simulink model "controller_dev_py"  (R2018b)
settings: Solver=ode2  StartTime=0.0  StopTime=inf  FixedStep=tS  RelTol=1e-3  EnableMultiTasking=on
model workspace (MAT data in the model file):
  m = 1000
settings Model: DataDictionary=controller_dev_py.sldd  PauseTimes=6.42  Creator=wischnewski  LastModifiedBy=ge34qer
settings DataIOCC: SaveOutput=off  SignalLogging=off  DSMLogging=off  SaveTime=off
settings OptimizationCC: StrengthReduction=on  PassReuseOutputArgsAs=Individual arguments  OptimizeBlockOrder=speed  OptimizationPriority=Speed  OptimizationCustomize=off
settings DebuggingCC: UnderspecifiedInitializationDetection=Classic  MergeDetectMultiDrivingBlocksExec=none  ParameterTunabilityLossMsg=error
settings ModelReferenceCC: PropagateSignalLabelsOutOfModel=off
settings SFSimCC: MATLABDynamicMemAlloc=off
settings RTWCC: SystemTargetFile=ert.tlc  GenCodeOnly=on  PackageGeneratedCodeAndArtifacts=on  PackageName=controller_dev_py  TemplateMakefile=ert_default_tmf  IncludeHyperlinkInReport=on  TargetLang=C++
settings CodeAppCC: ForceParamTrailComments=on  IgnoreCustomStorageClasses=off  MaxIdLength=64  OperatorAnnotations=on  SimulinkDataObjDesc=on  SFDataObjDesc=on  InsertBlockDesc=on
settings ERTTargetCC: TargetLangStandard=C++03 (ISO)  GenerateSampleERTMain=on  MultiInstanceERTCode=on  CodeInterfacePackaging=Reusable function  SupportContinuousTime=on  SupportVariableSizeSignals=on  GenerateAllocFcn=on  RootIOFormat=Part of model data structure  RTWCAPIParams=on  ERTCustomFileTemplate=example_file_process.tlc

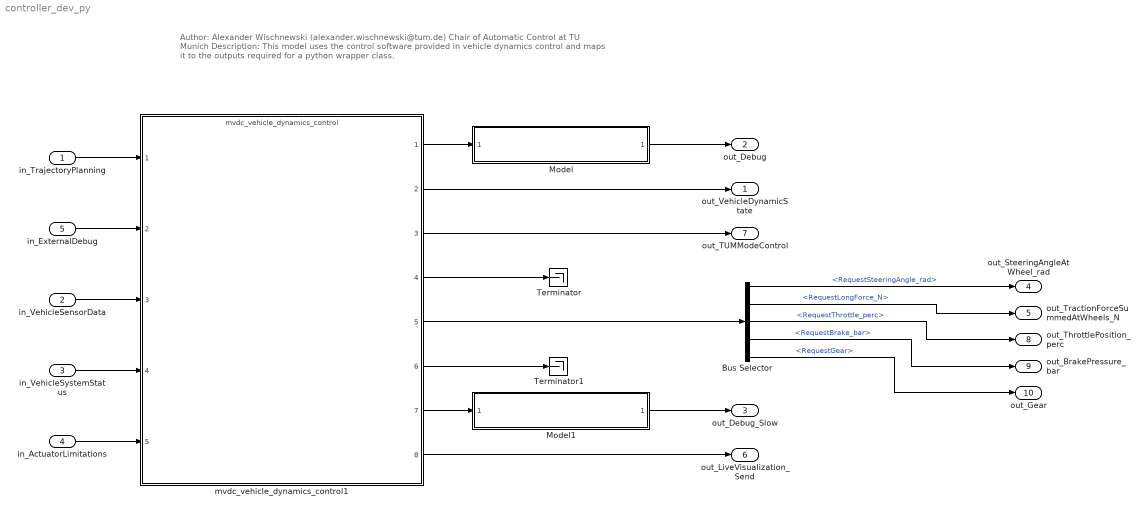
== system controller_dev_py ==
  note: Author: Alexander Wischnewski (alexander.wischnewski@tum.de)
      | Chair of Automatic Control at TU Munich
      |
      | Description: This model uses the control software provided in vehicle dynamics control and maps it to the outputs required for a python wrapper class.
  in_TrajectoryPlanning : Inport  OutDataTypeStr=Bus: TrajectoryPlanning
  in_VehicleSensorData : Inport  Port=2  OutDataTypeStr=Bus: VehicleSensorData
  in_VehicleSystemStatus : Inport  Port=3  OutDataTypeStr=Bus: VehicleSystemStatus
  in_ActuatorLimitations : Inport  Port=4  OutDataTypeStr=Bus: ActuatorLimitations
  in_ExternalDebug : Inport  Port=5  OutDataTypeStr=Bus: ExternalDebug
  Bus Selector : BusSelector  OutputSignals=RequestSteeringAngle_rad,RequestLongForce_N,RequestThrottle_perc,RequestBrake_bar,RequestGear
  Model : ModelReference  ModelNameDialog=debug_conversion_debug.slx  SimulationMode=Normal  ModelReferenceVersion=1.8
  Model1 : ModelReference  ModelNameDialog=debug_conversion_debug_slow.slx  SimulationMode=Normal  ModelReferenceVersion=1.8
  Terminator : Terminator
  Terminator1 : Terminator
  mvdc_vehicle_dynamics_control1 : ModelReference  ModelNameDialog=mvdc_vehicle_dynamics_control  SimulationMode=Normal  ModelReferenceVersion=1.801
  out_VehicleDynamicState : Outport  OutDataTypeStr=Bus: VehicleDynamicState
  out_Debug : Outport  Port=2
  out_Debug_Slow : Outport  Port=3
  out_SteeringAngleAtWheel_rad : Outport  Port=4
  out_TractionForceSummedAtWheels_N : Outport  Port=5
  out_LiveVisualization_Send : Outport  Port=6  OutDataTypeStr=Bus: LiveVisualization  PortDimensions=1  BusOutputAsStruct=on
  out_TUMModeControl : Outport  Port=7  OutDataTypeStr=Bus: TUMModeControl
  out_ThrottlePosition_perc : Outport  Port=8
  out_BrakePressure_bar : Outport  Port=9
  out_Gear : Outport  Port=10
  wires:
  in_TrajectoryPlanning/1 -> mvdc_vehicle_dynamics_control1/1
  mvdc_vehicle_dynamics_control1/2 -> out_VehicleDynamicState/1
  Model/1 -> out_Debug/1
  mvdc_vehicle_dynamics_control1/1 -> Model/1
  mvdc_vehicle_dynamics_control1/7 -> Model1/1
  Model1/1 -> out_Debug_Slow/1
  in_VehicleSensorData/1 -> mvdc_vehicle_dynamics_control1/3
  in_VehicleSystemStatus/1 -> mvdc_vehicle_dynamics_control1/4
  in_ActuatorLimitations/1 -> mvdc_vehicle_dynamics_control1/5
  mvdc_vehicle_dynamics_control1/4 -> Terminator/1
  mvdc_vehicle_dynamics_control1/6 -> Terminator1/1
  mvdc_vehicle_dynamics_control1/5 -> Bus Selector/1
  Bus Selector/1 -> out_SteeringAngleAtWheel_rad/1  "<RequestSteeringAngle_rad>"
  Bus Selector/2 -> out_TractionForceSummedAtWheels_N/1  "<RequestLongForce_N>"
  mvdc_vehicle_dynamics_control1/8 -> out_LiveVisualization_Send/1
  mvdc_vehicle_dynamics_control1/3 -> out_TUMModeControl/1
  Bus Selector/3 -> out_ThrottlePosition_perc/1  "<RequestThrottle_perc>"
  Bus Selector/4 -> out_BrakePressure_bar/1  "<RequestBrake_bar>"
  Bus Selector/5 -> out_Gear/1  "<RequestGear>"
  in_ExternalDebug/1 -> mvdc_vehicle_dynamics_control1/2
